simulink model "test_atrias_hip"  (R2014b)
settings: Solver=FixedStepDiscrete  StartTime=0.0  StopTime=inf  FixedStep=0.001  RelTol=1e-3
StartFcn:
  | tg.sampletime = correctedSampleTime;
libraries: xpcethercatlib x6, slrtlib x5, simulink x1
settings Model: SimulationMode=external  BufferReuse=off  Creator=drl  LastModifiedBy=drl
settings SolverCC: EnableConcurrentExecution=on  ConcurrentTasks=on
settings OptimizationCC: BlockReduction=off  OptimizeBlockIOStorage=off  BufferReuse=off  GlobalBufferReuse=off  ExpressionFolding=off  LocalBlockOutputs=off
settings HardwareCC: ProdIntDivRoundTo=Zero  ProdEndianess=LittleEndian  ProdLongLongMode=on  ProdHWDeviceType=Generic->32-bit x86 compatible
settings RTWCC: SystemTargetFile=slrt.tlc  TemplateMakefile=slrt_default_tmf  Description=Simulink Real-Time  ProcessScript=slrt_make_rtw_hook  RTWCompilerOptimization=On
settings SimulinkRealTimeCC: GeneratePreprocessorConditionals=Disable all  EnableShiftOperators=on

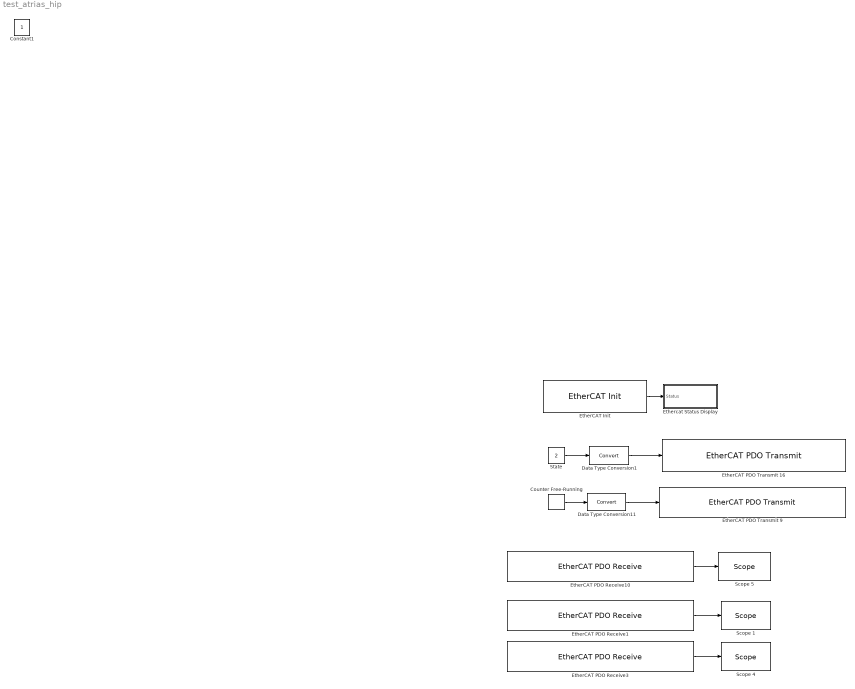
== system test_atrias_hip ==
  Counter Free-Running : simulink/Sources/Counter Free-Running  NumBits=16  tsamp=-1
  Data Type Conversion1 : DataTypeConversion
  Data Type Conversion11 : DataTypeConversion
  "EtherCAT Init " : xpcethercatlib/EtherCAT Init   Priority=0  config_file=hipMedulla_eni.xml  device_id=0  pci_bus=2  pci_slot=0  enaDebug=off  enaDC=on  errLink=off  masterDbg=off  stateChgDbg=off  baseClock=off  masterCfg=off  logFile='c:\dbglog.txt'  sample_time=0.001000
  EtherCAT PDO Receive1 : xpcethercatlib/EtherCAT PDO Receive  Priority=2  sig_name=Box 1 (ATRIAS 2.1 Hip (Medulla 1.5)).Hip Encoder.Encoder  sig_offset=504  sig_type=uint32  type_size=32  sig_dim=1  device_id=0  sample_time=0.001000
  EtherCAT PDO Receive10 : xpcethercatlib/EtherCAT PDO Receive  Priority=2  sig_name=Box 1 (ATRIAS 2.1 Hip (Medulla 1.5)).uController Status.State  sig_offset=472  sig_type=uint8  type_size=8  sig_dim=1  device_id=0  sample_time=0.001000
  EtherCAT PDO Receive3 : xpcethercatlib/EtherCAT PDO Receive  Priority=2  sig_name=Box 1 (ATRIAS 2.1 Hip (Medulla 1.5)).uController Status.Counter  sig_offset=480  sig_type=uint8  type_size=8  sig_dim=1  device_id=0  sample_time=0.001000
  EtherCAT PDO Transmit 16 : xpcethercatlib/EtherCAT PDO Transmit   Priority=3  sig_name=Box 1 (ATRIAS 2.1 Hip (Medulla 1.5)).uControllerInput.Command  sig_offset=464  sig_type=uint8  type_size=8  sig_dim=1  device_id=0  sample_time=0.001000
  EtherCAT PDO Transmit 9 : xpcethercatlib/EtherCAT PDO Transmit   Priority=3  sig_name=Box 1 (ATRIAS 2.1 Hip (Medulla 1.5)).uControllerInput.Counter  sig_offset=472  sig_type=uint16  type_size=16  sig_dim=1  device_id=0  sample_time=0.001000
  Ethercat Status Display : Subsystem
  Scope 1 : slrtlib/Displays and Logging/Scope   scopeno=1  scopetype=Target  autostart=on  viewmode=Graphical sliding  formatstr='%f'  grid=on  ylimits=[0,0]  nosamples=10000  noprepostsamples=0  interleave=1  triggermode=FreeRun  triggersignal=1  trigsignalfromport=off  triggerlevel=0.0  triggerslope=Either  triggerscope=1  triggersample=0  filename=data.dat  mode=Lazy  writesize=512  autorestart=off  dynamicfilemode=off  maxwritefilesize=512*1024^2
  Scope 4 : slrtlib/Displays and Logging/Scope   scopeno=9  scopetype=Target  autostart=on  viewmode=Graphical sliding  formatstr='%f'  grid=on  ylimits=[0,0]  nosamples=10000  noprepostsamples=0  interleave=1  triggermode=FreeRun  triggersignal=1  trigsignalfromport=off  triggerlevel=0.0  triggerslope=Either  triggerscope=1  triggersample=0  filename=data.dat  mode=Lazy  writesize=512  autorestart=off  dynamicfilemode=off  maxwritefilesize=512*1024^2
  Scope 5 : slrtlib/Displays and Logging/Scope   scopeno=7  scopetype=Target  autostart=on  viewmode=Numerical  formatstr='%f'  grid=on  ylimits=[0,0]  nosamples=100  noprepostsamples=0  interleave=1  triggermode=FreeRun  triggersignal=1  trigsignalfromport=off  triggerlevel=0.0  triggerslope=Either  triggerscope=1  triggersample=0  filename=data.dat  mode=Lazy  writesize=512  autorestart=off  dynamicfilemode=off  maxwritefilesize=512*1024^2
  State : Constant  Value=2
  Constant1 : Constant  IOType=siggen
  wires:
  "EtherCAT Init "/1 -> Ethercat Status Display/1(Status)
  EtherCAT PDO Receive3/1 -> Scope 4/1
  EtherCAT PDO Receive1/1 -> Scope 1/1
  EtherCAT PDO Receive10/1 -> Scope 5/1
  Data Type Conversion11/1 -> EtherCAT PDO Transmit 9/1
  Counter Free-Running/1 -> Data Type Conversion11/1
  State/1 -> Data Type Conversion1/1
  Data Type Conversion1/1 -> EtherCAT PDO Transmit 16/1

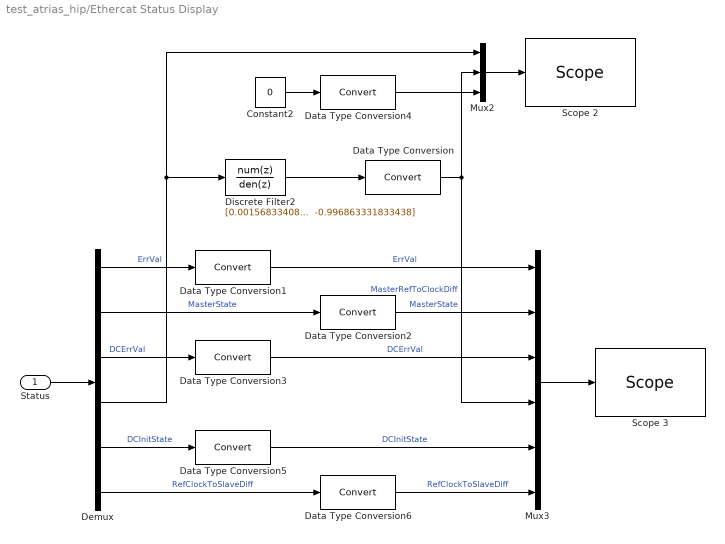
== system test_atrias_hip/Ethercat Status Display ==
  Status : Inport
  Constant2 : Constant  Value=0  OutDataTypeStr=Inherit: Inherit via back propagation  SampleTime=-1
  Data Type Conversion{,1..6} (7 alike) : DataTypeConversion
  Demux : Demux  Outputs=6
  Discrete Filter2 : DiscreteFilter  Numerator="[0.001568334083281   0.001568334083281]"  Denominator="[1.000000000000000  -0.996863331833438]"  a0EqualsOne=on
  Mux2 : Mux  Inputs=3
  Mux3 : Mux  Inputs=6
  Scope 2 : slrtlib/Displays and Logging/Scope   scopeno=5  scopetype=Target  autostart=on  viewmode=Graphical rolling  formatstr='%f'  grid=on  ylimits=[0,0]  nosamples=10000  noprepostsamples=0  interleave=1  triggermode=FreeRun  triggersignal=1  trigsignalfromport=off  triggerlevel=0.0  triggerslope=Either  triggerscope=1  triggersample=0  filename=data.dat  mode=Lazy  writesize=512  autorestart=off  dynamicfilemode=off  maxwritefilesize=512*1024^2
  Scope 3 : slrtlib/Displays and Logging/Scope   scopeno=6  scopetype=Target  autostart=on  viewmode=Numerical  formatstr='%15.6f'  grid=on  ylimits=[0,0]  nosamples=100  noprepostsamples=0  interleave=1  triggermode=FreeRun  triggersignal=1  trigsignalfromport=off  triggerlevel=0.0  triggerslope=Either  triggerscope=1  triggersample=0  filename=data.dat  mode=Lazy  writesize=512  autorestart=off  dynamicfilemode=off  maxwritefilesize=512*1024^2
  wires:
  Status/1 -> Demux/1
  Demux/4 -> Discrete Filter2/1, Mux2/1
  Discrete Filter2/1 -> Data Type Conversion/1
  Mux2/1 -> Scope 2/1
  Constant2/1 -> Data Type Conversion4/1
  Data Type Conversion4/1 -> Mux2/3
  Mux3/1 -> Scope 3/1
  Data Type Conversion/1 -> Mux3/4, Mux2/2  "MasterRefToClockDiff"
  Data Type Conversion1/1 -> Mux3/1  "ErrVal"
  Data Type Conversion2/1 -> Mux3/2  "MasterState"
  Data Type Conversion3/1 -> Mux3/3  "DCErrVal"
  Data Type Conversion5/1 -> Mux3/5  "DCInitState"
  Data Type Conversion6/1 -> Mux3/6  "RefClockToSlaveDiff"
  Demux/1 -> Data Type Conversion1/1  "ErrVal"
  Demux/2 -> Data Type Conversion2/1  "MasterState"
  Demux/3 -> Data Type Conversion3/1  "DCErrVal"
  Demux/5 -> Data Type Conversion5/1  "DCInitState"
  Demux/6 -> Data Type Conversion6/1  "RefClockToSlaveDiff"
